simulink model "visualmodel"  (R2023b)
settings: Solver=VariableStepAuto  StartTime=0.0  StopTime=10.0  RelTol=1e-3
values from neighbouring files (symbols this model uses):
  G = [0 0 0     0 0 0    0 0 0    0 0 0]'    [hopsim1.m]    (also in hopsim2.m = [0 0   0 0   0 0 10    0 0 0]')
  K = round(K,5)    [hopsim1.m]    (also in hopsim2.m)
libraries: shared6dof x1
settings Model: Creator=jacksonwright  LastModifiedBy=jacksonwright

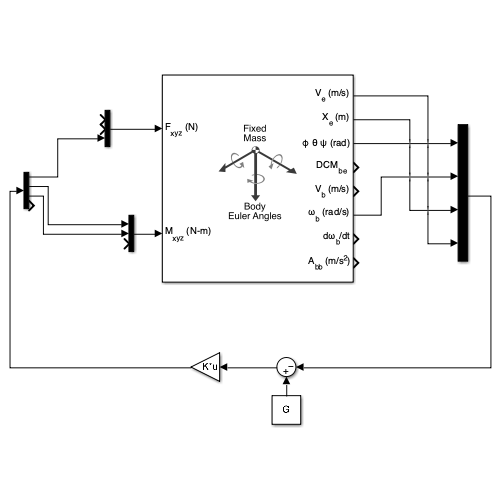
[thumbnail: Simulink's stored preview of the top-level diagram]
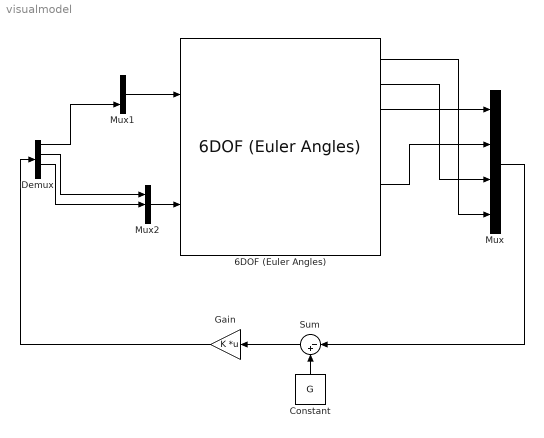
== system visualmodel ==
  6DOF (Euler Angles) : shared6dof/6DOF (Euler Angles)  units=Metric (MKS)  mtype=Fixed  rep=Euler Angles  xme_0=[0 0 0]  Vm_0=[0 0 0]  eul_0=[0 0 0]  pm_0=[0 0 0]  mass_0=1.0  mass_e=0.5  mass_f=2.0  inertia=eye(3)  inertia_e=eye(3)  inertia_f=2*eye(3)  k_quat=1.0  vre_flag=on  abi_flag=off  aMode=0  xme_statename=''  Vm_statename=''  eul_statename=''  quat_statename=''  pm_statename=''  mass_statename=''
  Constant : Constant  Value=G
  Demux : Demux
  Gain : Gain  Gain=K  Multiplication=Matrix(K*u)
  Mux : Mux
  Mux1 : Mux  Inputs=3
  Mux2 : Mux  Inputs=3
  Sum : Sum  Inputs=|-+
  wires:
  6DOF (Euler Angles)/3 -> Mux/1
  6DOF (Euler Angles)/6 -> Mux/2
  6DOF (Euler Angles)/2 -> Mux/3
  6DOF (Euler Angles)/1 -> Mux/4
  Mux/1 -> Sum/1
  Constant/1 -> Sum/2
  Sum/1 -> Gain/1
  Gain/1 -> Demux/1
  Demux/1 -> Mux1/3
  Mux1/1 -> 6DOF (Euler Angles)/1
  Demux/2 -> Mux2/1
  Demux/3 -> Mux2/2
  Mux2/1 -> 6DOF (Euler Angles)/2
